simulink model "Models_P"  (R2019b)
settings: Solver=FixedStepAuto  StartTime=0.0  StopTime=10  RelTol=1e-3
values from neighbouring files (symbols this model uses):
  Parameters = struct('m1', m1, 'l1', l1, 'm2', m2, 'l2', l2, 'I2', I2, 'Kf2', Kf2, 'g', g, 'Km', Km, 'Rm', Rm, 'Jm', Jm, 'bm', bm, 'x1', x1, 'x2', x2)    [FitParameters.m]
undefined symbols (not defined in the file or in its folder): tf2_1, tf2_2
libraries: simulink x1
settings Model: Creator=Guido  LastModifiedBy=pietr
settings DataIOCC: SignalLogging=off  DSMLogging=off  InspectSignalLogs=on  ReturnWorkspaceOutputs=off

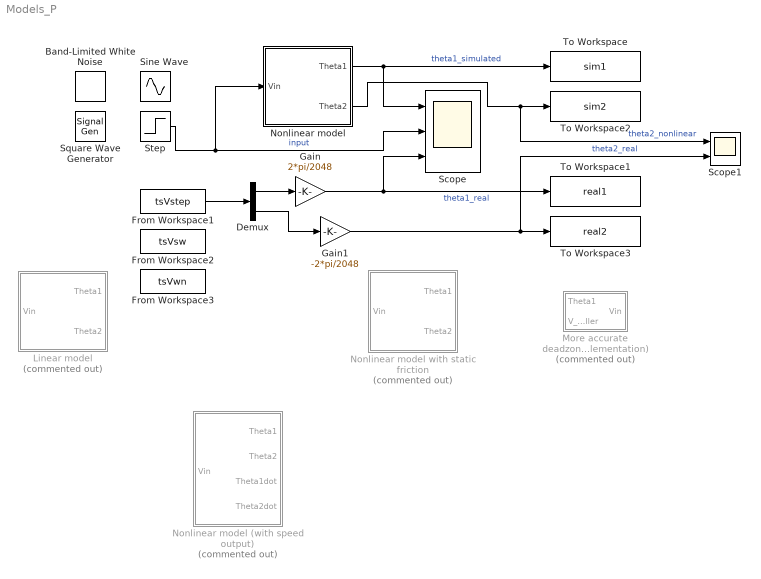
== system Models_P ==
  Band-Limited White Noise : simulink/Sources/Band-Limited White Noise  Cov=[0.1]  Ts=0.1  seed=[23341]
  Demux : Demux  Outputs=2
  From Workspace1 : FromWorkspace  VariableName=tsVstep  SampleTime=0
  From Workspace2 : FromWorkspace  VariableName=tsVsw  SampleTime=0
  From Workspace3 : FromWorkspace  VariableName=tsVwn  SampleTime=0
  Gain : Gain  Gain=2*pi/2048
  Gain1 : Gain  Gain=-2*pi/2048
  Linear model : Subsystem  Commented=on
  More accurate deadzone (Alternative friction implementation) : Subsystem  Commented=on
  Nonlinear model : Subsystem
  Nonlinear model (with speed output) : Subsystem  Commented=on
  Nonlinear model with static friction : Subsystem  Commented=on
  Scope : Scope  NumInputPorts=3
  Scope1 : Scope  NumInputPorts=2
  Sine Wave : Sin  Frequency=11  SampleTime=0
  Square Wave Generator : SignalGenerator  WaveForm=square
  Step : Step  After=0.8  SampleTime=0
  To Workspace : ToWorkspace  VariableName=sim1  SampleTime=-1
      settings: Save2DSignal=2-D array (concatenate along first dimension)
  To Workspace1 : ToWorkspace  VariableName=real1  SampleTime=-1
      settings: Save2DSignal=2-D array (concatenate along first dimension)
  To Workspace2 : ToWorkspace  VariableName=sim2  SampleTime=-1
      settings: Save2DSignal=2-D array (concatenate along first dimension)
  To Workspace3 : ToWorkspace  VariableName=real2  SampleTime=-1
      settings: Save2DSignal=2-D array (concatenate along first dimension)
  wires:
  Nonlinear model/1(Theta1) -> To Workspace/1, Scope/1  "theta1_simulated"
  Gain/1 -> To Workspace1/1, Scope/3  "theta1_real"
  Demux/1 -> Gain/1
  Step/1 -> Scope/2, Nonlinear model/1(Vin)  "input"
  Demux/2 -> Gain1/1
  Gain1/1 -> Scope1/2, To Workspace3/1  "theta2_real"
  Nonlinear model/2(Theta2) -> Scope1/1, To Workspace2/1  "theta2_nonlinear"
  From Workspace1/1 -> Demux/1

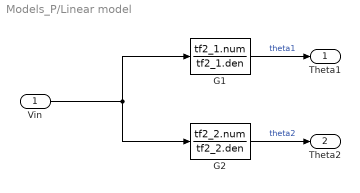
== system Models_P/Linear model ==
  Vin : Inport
  G1 : TransferFcn  Numerator=tf2_1.num  Denominator=tf2_1.den
  G2 : TransferFcn  Numerator=tf2_2.num  Denominator=tf2_2.den
  Theta1 : Outport
  Theta2 : Outport  Port=2
  wires:
  Vin/1 -> G2/1, G1/1
  G1/1 -> Theta1/1  "theta1"
  G2/1 -> Theta2/1  "theta2"

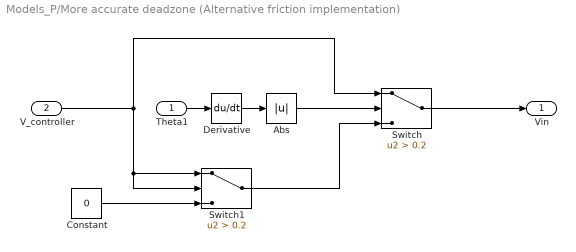
== system Models_P/More accurate deadzone (Alternative friction implementation) ==
  Theta1 : Inport
  V_controller : Inport  Port=2
  Abs : Abs
  Constant : Constant  Value=0
  Derivative : Derivative
  Switch : Switch  Criteria=u2 > Threshold  Threshold=0.2
  Switch1 : Switch  Criteria=u2 > Threshold  Threshold=0.2
  Vin : Outport
  wires:
  V_controller/1 -> Switch1/2, Switch1/1, Switch/1
  Theta1/1 -> Derivative/1
  Derivative/1 -> Abs/1
  Switch/1 -> Vin/1
  Abs/1 -> Switch/2
  Switch1/1 -> Switch/3
  Constant/1 -> Switch1/3

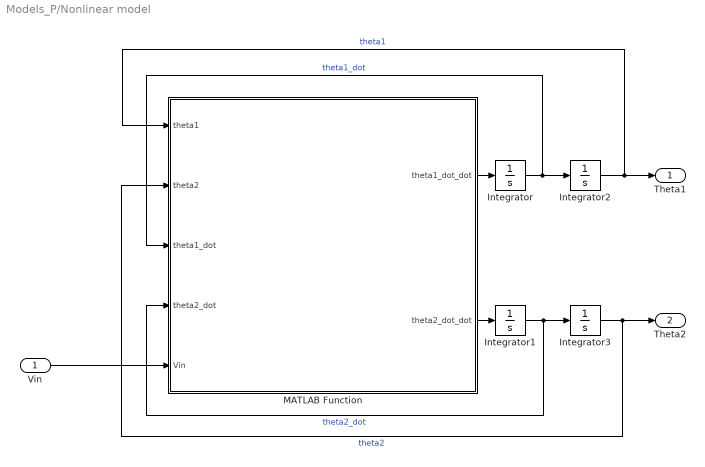
== system Models_P/Nonlinear model ==
  Vin : Inport
  Integrator{,1..3} (4 alike) : Integrator
  MATLAB Function : MATLAB Function  TreatAsAtomicUnit=on  mask{Pars=Parameters}
      mask prompts: Pars "Struct containing model parameters"
  Theta1 : Outport
  Theta2 : Outport  Port=2
  wires:
  Integrator/1 -> MATLAB Function/3(theta1_dot), Integrator2/1  "theta1_dot"
  Integrator1/1 -> MATLAB Function/4(theta2_dot), Integrator3/1  "theta2_dot"
  MATLAB Function/1(theta1_dot_dot) -> Integrator/1
  Integrator3/1 -> Theta2/1, MATLAB Function/2(theta2)  "theta2"
  MATLAB Function/2(theta2_dot_dot) -> Integrator1/1
  Integrator2/1 -> MATLAB Function/1(theta1), Theta1/1  "theta1"
  Vin/1 -> MATLAB Function/5(Vin)

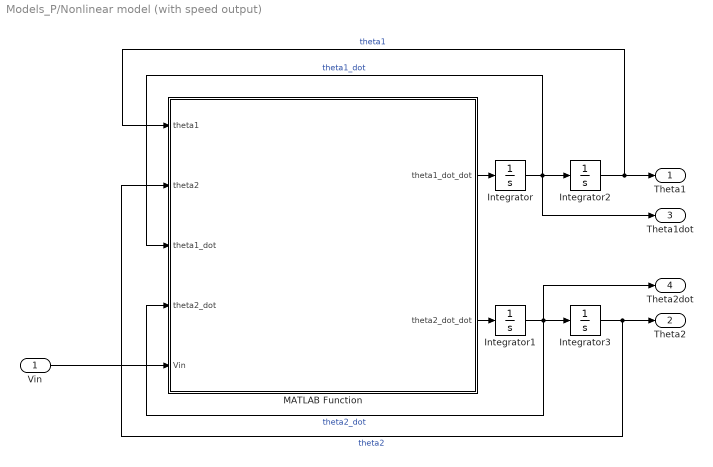
== system Models_P/Nonlinear model (with speed output) ==
  Vin : Inport
  Integrator{,1..3} (4 alike) : Integrator
  MATLAB Function : MATLAB Function  TreatAsAtomicUnit=on  mask{Pars=Parameters}
      mask prompts: Pars "Struct containing model parameters"
  Theta1 : Outport
  Theta2 : Outport  Port=2
  Theta1dot : Outport  Port=3
  Theta2dot : Outport  Port=4
  wires:
  Integrator/1 -> Theta1dot/1, MATLAB Function/3(theta1_dot), Integrator2/1  "theta1_dot"
  Integrator1/1 -> Theta2dot/1, MATLAB Function/4(theta2_dot), Integrator3/1  "theta2_dot"
  MATLAB Function/1(theta1_dot_dot) -> Integrator/1
  Integrator3/1 -> Theta2/1, MATLAB Function/2(theta2)  "theta2"
  MATLAB Function/2(theta2_dot_dot) -> Integrator1/1
  Integrator2/1 -> MATLAB Function/1(theta1), Theta1/1  "theta1"
  Vin/1 -> MATLAB Function/5(Vin)

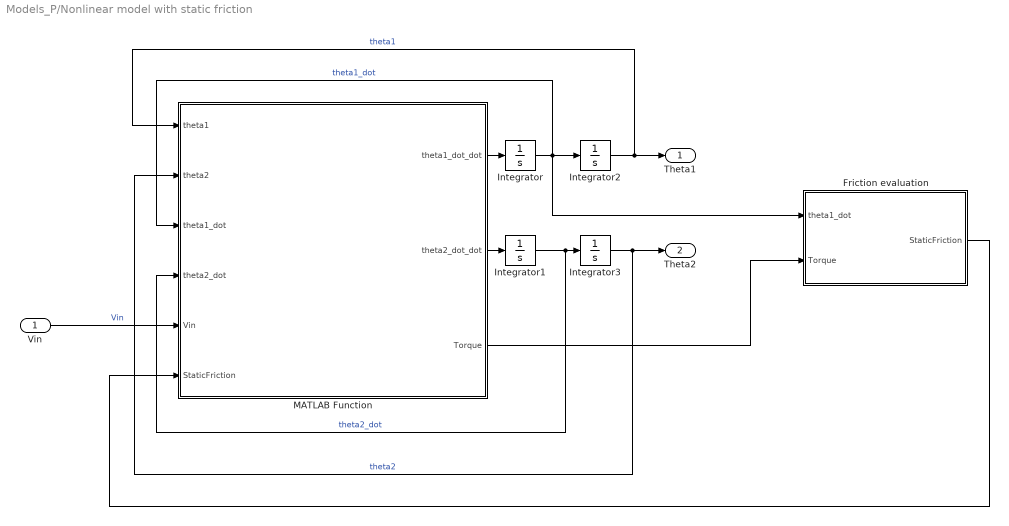
== system Models_P/Nonlinear model with static friction ==
  Vin : Inport
  Friction evaluation : MATLAB Function  TreatAsAtomicUnit=on  mask{Pars=Parameters, AlmostZeroSpeed=1, DeadzoneSensitivity=0.2}
      mask prompts: Pars "Parameters struct (Do not change!)"; AlmostZeroSpeed "Speed under which the Static friction comes into play"; DeadzoneSensitivity "Value of input voltage needed to win static friction"
  Integrator{,1..3} (4 alike) : Integrator
  MATLAB Function : MATLAB Function  TreatAsAtomicUnit=on  mask{Pars=Parameters}
      mask prompts: Pars "Struct containing model parameters"
  Theta1 : Outport
  Theta2 : Outport  Port=2
  wires:
  Integrator/1 -> Friction evaluation/1(theta1_dot), Integrator2/1, MATLAB Function/3(theta1_dot)  "theta1_dot"
  Integrator1/1 -> MATLAB Function/4(theta2_dot), Integrator3/1  "theta2_dot"
  MATLAB Function/1(theta1_dot_dot) -> Integrator/1
  Integrator3/1 -> MATLAB Function/2(theta2), Theta2/1  "theta2"
  MATLAB Function/2(theta2_dot_dot) -> Integrator1/1
  Integrator2/1 -> Theta1/1, MATLAB Function/1(theta1)  "theta1"
  Vin/1 -> MATLAB Function/5(Vin)  "Vin"
  MATLAB Function/3(Torque) -> Friction evaluation/2(Torque)
  Friction evaluation/1(StaticFriction) -> MATLAB Function/6(StaticFriction)

== matlab function Models_P/Nonlinear model with static friction/Friction evaluation ==
  data: theta1_dot input; Torque input; StaticFriction output; Pars parameter; DeadzoneSensitivity parameter; AlmostZeroSpeed parameter
function StaticFriction = fcn(theta1_dot, Torque, Pars, DeadzoneSensitivity, AlmostZeroSpeed)

%the static friction has a maximum value, then decreases towards 0 as the
%speed approaches AlmostZeroSpeed. After it is zero.
if abs(theta1_dot) <= AlmostZeroSpeed 
    MaxFriction = min(Torque, Pars.Km/Pars.Rm*(DeadzoneSensitivity-Pars.Km*theta1_dot));
    MaxFriction = max(MaxFriction, 0); %To ensure the friction is not negative
    StaticFriction = MaxFriction*(AlmostZeroSpeed-abs(theta1_dot)); %MaxFriction weighted by the speed difference
else
    StaticFriction = 0;
end

== matlab function Models_P/Nonlinear model/MATLAB Function ==
  data: theta1 input; theta1_dot_dot output; theta2 input; theta1_dot input; theta2_dot input; Vin input; theta2_dot_dot output; Pars parameter
function [theta1_dot_dot,theta2_dot_dot] = fcn(theta1, theta2, theta1_dot, theta2_dot,Vin, Pars)

   k1 = Pars.Jeq + Pars.m2*(Pars.l1^2 + Pars.x2^2*sin(theta2)^2);
   k2 = Pars.m2*Pars.l1*Pars.x2*cos(theta2);
   k3 = 2*Pars.m2*Pars.x2^2*sin(theta2)*cos(theta2)*theta1_dot*theta2_dot - Pars.m2*Pars.l1*Pars.x2*sin(theta2)*theta2_dot^2 +Pars.Ks*theta1 - Pars.Km/Pars.Rm*Vin + (Pars.Km^2)/Pars.Rm*theta1_dot + Pars.Kf1*theta1_dot;
   k4 = Pars.m2*Pars.l1*Pars.x2*cos(theta2);
   k5 = Pars.m2*Pars.x2^2 + Pars.I2;
   k6 = - Pars.m2*Pars.x2^2*sin(theta2)*cos(theta2)*theta1_dot^2 + Pars.m2*Pars.g*Pars.x2*sin(theta2) + Pars.Kf2*theta2_dot;


theta1_dot_dot = (k2*k6 - k3*k5)/(k1*k5 - k2*k4);
theta2_dot_dot = -(k1*k6 - k3*k4)/(k1*k5 - k2*k4);

== matlab function Models_P/Nonlinear model with static friction/MATLAB Function ==
  data: theta1 input; theta1_dot_dot output; theta2_dot_dot output; Torque output; theta2 input; theta1_dot input; theta2_dot input; Vin input; StaticFriction input; Pars parameter
function [theta1_dot_dot, theta2_dot_dot, Torque] = fcn(theta1, theta2, theta1_dot, theta2_dot, Vin, StaticFriction, Pars)

   k1 = Pars.Jeq + Pars.m2*(Pars.l1^2 + Pars.x2^2*sin(theta2)^2);
   k2 = Pars.m2*Pars.l1*Pars.x2*cos(theta2);
   k3 = 2*Pars.m2*Pars.x2^2*sin(theta2)*cos(theta2)*theta1_dot*theta2_dot - Pars.m2*Pars.l1*Pars.x2*sin(theta2)*theta2_dot^2 +Pars.Ks*theta1 - Pars.Km/Pars.Rm*Vin + (Pars.Km^2)/Pars.Rm*theta1_dot + Pars.Kf1*theta1_dot + StaticFriction;
   k4 = Pars.m2*Pars.l1*Pars.x2*cos(theta2);
   k5 = Pars.m2*Pars.x2^2 + Pars.I2;
   k6 = - Pars.m2*Pars.x2^2*sin(theta2)*cos(theta2)*theta1_dot^2 + Pars.m2*Pars.g*Pars.x2*sin(theta2) + Pars.Kf2*theta2_dot;


theta1_dot_dot = (k2*k6 - k3*k5)/(k1*k5 - k2*k4);
theta2_dot_dot = -(k1*k6 - k3*k4)/(k1*k5 - k2*k4);
Torque = Pars.Km/Pars.Rm*(Vin-Pars.Km*theta1_dot);

== matlab function Models_P/Nonlinear model (with speed output)/MATLAB Function ==
  data: theta1 input; theta1_dot_dot output; theta2 input; theta1_dot input; theta2_dot input; Vin input; theta2_dot_dot output; Pars parameter
function [theta1_dot_dot,theta2_dot_dot] = fcn(theta1, theta2, theta1_dot, theta2_dot,Vin, Pars)

   k1 = Pars.Jeq + Pars.m2*(Pars.l1^2 + Pars.x2^2*sin(theta2)^2);
   k2 = Pars.m2*Pars.l1*Pars.x2*cos(theta2);
   k3 = 2*Pars.m2*Pars.x2^2*sin(theta2)*cos(theta2)*theta1_dot*theta2_dot - Pars.m2*Pars.l1*Pars.x2*sin(theta2)*theta2_dot^2 +Pars.Ks*theta1 - Pars.Km/Pars.Rm*Vin + (Pars.Km^2)/Pars.Rm*theta1_dot + Pars.Kf1*theta1_dot;
   k4 = Pars.m2*Pars.l1*Pars.x2*cos(theta2);
   k5 = Pars.m2*Pars.x2^2 + Pars.I2;
   k6 = - Pars.m2*Pars.x2^2*sin(theta2)*cos(theta2)*theta1_dot^2 + Pars.m2*Pars.g*Pars.x2*sin(theta2) + Pars.Kf2*theta2_dot;


theta1_dot_dot = (k2*k6 - k3*k5)/(k1*k5 - k2*k4);
theta2_dot_dot = -(k1*k6 - k3*k4)/(k1*k5 - k2*k4);
